simulink subsystem "myTHD"  (R2024a)
settings: Solver=VariableStepAuto  StartTime=0.0  StopTime=10.0  RelTol=1e-3
libraries: embmathops x1, hdlsllib x1
settings Model: Creator=Jan Rosa  LastModifiedBy=Jan Rosa

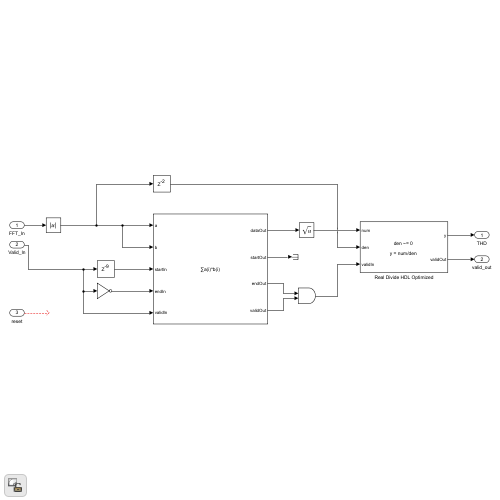
[thumbnail: Simulink's stored preview of the top-level diagram]
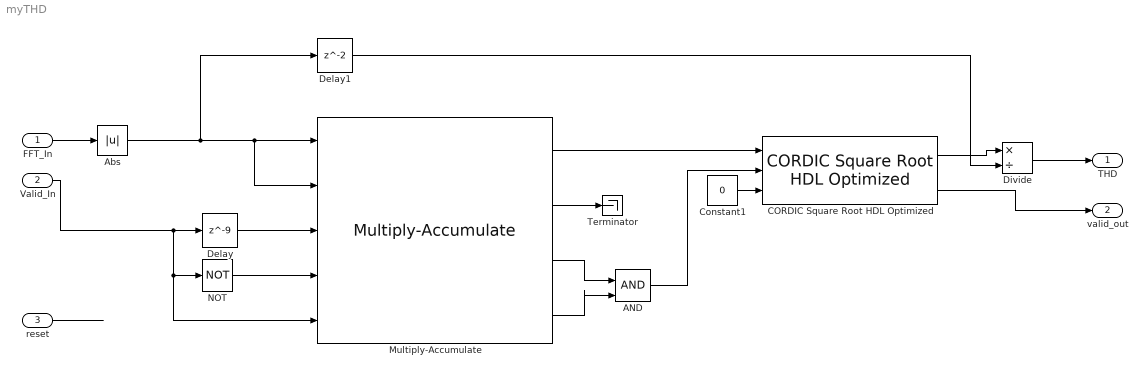
== system myTHD ==
  FFT_In : Inport
  Valid_In : Inport  Port=2
  reset : Inport  Port=3
  AND : Logic  IconShape=distinctive  AllPortsSameDT=off  OutDataTypeStr=boolean
  Abs : Abs  SaturateOnIntegerOverflow=off
  CORDIC Square Root HDL Optimized : embmathops/CORDIC Square Root HDL Optimized  autoMaximumShiftVal=on  maximumShiftValue=10  nIterPerReg=1
      settings: LibrarySourceBlock=embeddedMatrixLib/Math Operations/CORDIC Square Root HDL Optimized
  Constant1 : Constant  Value=0
  Delay : Delay  DelayLength=9
  Delay1 : Delay
  Divide : Product  Inputs=*/
  Multiply-Accumulate : hdlsllib/HDL Operations/Multiply-Accumulate  opMode=Streaming - using Start and End ports  initValueSetting=Dialog  initValue=0  initValueSetting2=Dialog  initValue2=0  initValueSetting3=Dialog  initValue3=0  num_samples=2  RndMeth2=Floor  RndMeth3=Floor  datatype2=Inherit: Inherit via back propagation  datatype3=Inherit: Inherit via back propagation  validOut=on  endInandOut=on  startOut=on  countOut=on  dim=-1  DoSatur=off  parallel=off
  NOT : Logic  Operator=NOT  IconShape=distinctive  AllPortsSameDT=off  OutDataTypeStr=boolean
  Terminator : Terminator
  THD : Outport
  valid_out : Outport  Port=2
  wires:
  FFT_In/1 -> Abs/1
  reset/1 -> ?
  Abs/1 -> Multiply-Accumulate/1, Multiply-Accumulate/2, Delay1/1
  Delay/1 -> Multiply-Accumulate/3
  NOT/1 -> Multiply-Accumulate/4
  Multiply-Accumulate/2 -> Terminator/1
  Valid_In/1 -> Delay/1, Multiply-Accumulate/5, NOT/1
  Multiply-Accumulate/1 -> CORDIC Square Root HDL Optimized/1
  Multiply-Accumulate/3 -> AND/1
  Multiply-Accumulate/4 -> AND/2
  AND/1 -> CORDIC Square Root HDL Optimized/2
  Delay1/1 -> Divide/2
  Divide/1 -> THD/1
  CORDIC Square Root HDL Optimized/2 -> valid_out/1
  Constant1/1 -> CORDIC Square Root HDL Optimized/3
  CORDIC Square Root HDL Optimized/1 -> Divide/1
